simulink model "Transformation_dq_alphabeta_123_V1"  (R2022a)
settings: Solver=VariableStepAuto  StartTime=0.0  StopTime=0.2  RelTol=1e-3
InitFcn:
  | Ts_xadc = 0.1;
values from neighbouring files (symbols this model uses):
  f_c = 100000    [Trans_dq_alphabeta_123_params.m]
  T_50MHz = 1/f_50MHz    (= 2e-08)    [Trans_dq_alphabeta_123_params.m]
libraries: simulink x3
settings Model: DataTypeOverride=Off  Creator=trichte  LastModifiedBy=Andre Merx
settings SolverCC: AlgebraicLoopSolver=TrustRegion
settings DataIOCC: LimitDataPoints=on  SaveFormat=Array  SaveOutput=off  SaveTime=off  ReturnWorkspaceOutputs=off
settings OptimizationCC: BlockReduction=off  ConditionallyExecuteInputs=off  DefaultParameterBehavior=Inlined  LifeSpan=inf
settings DebuggingCC: AlgebraicLoopMsg=error  SolverPrmCheckMsg=warning  UnconnectedInputMsg=warning  UnconnectedOutputMsg=warning  UnconnectedLineMsg=warning  AllowSymbolicDim=off  StrictBusMsg=ErrorOnBusTreatedAsVector  SFUnexpectedBacktrackingDiag=warning  SFNoUnconditionalDefaultTransitionDiag=warning  SFExecutionAtInitializationDiag=none  SFMachineParentedDataDiag=warning  ArithmeticOperatorsInVariantConditions=warning
settings HardwareCC: ProdBitPerPointer=32  ProdBitPerSizeT=32  ProdBitPerPtrDiffT=32  ProdLargestAtomicFloat=None  ProdIntDivRoundTo=Undefined  ProdEndianess=Unspecified  ProdWordSize=32  ProdHWDeviceType=ASIC/FPGA->ASIC/FPGA  ProdEqTarget=off
settings ModelReferenceCC: PropagateSignalLabelsOutOfModel=off
settings SFSimCC: SimUseLocalCustomCode=off  CustomCodeUndefinedFunction=UseInterfaceOnly
settings RTWCC: RTWUseLocalCustomCode=off
settings CodeAppCC: StateflowObjectComments=on
settings GRTTargetCC: TargetLangStandard=C89/C90 (ANSI)
settings ConfigComp: CovMetricSettings=dw  CovSaveCumulativeToWorkspaceVar=on  CovSaveSingleToWorkspaceVar=on  CovExternalEMLEnable=off  CovSFcnEnable=off

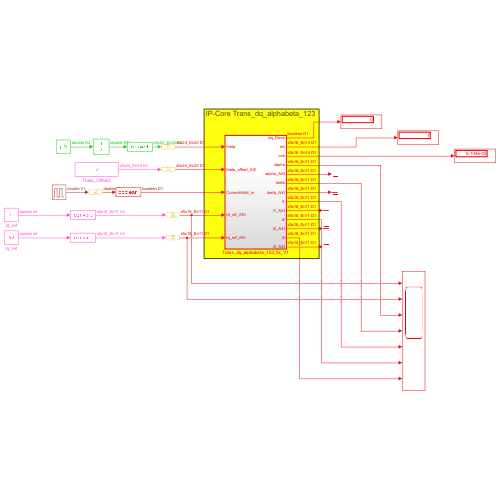
[thumbnail: Simulink's stored preview of the top-level diagram]
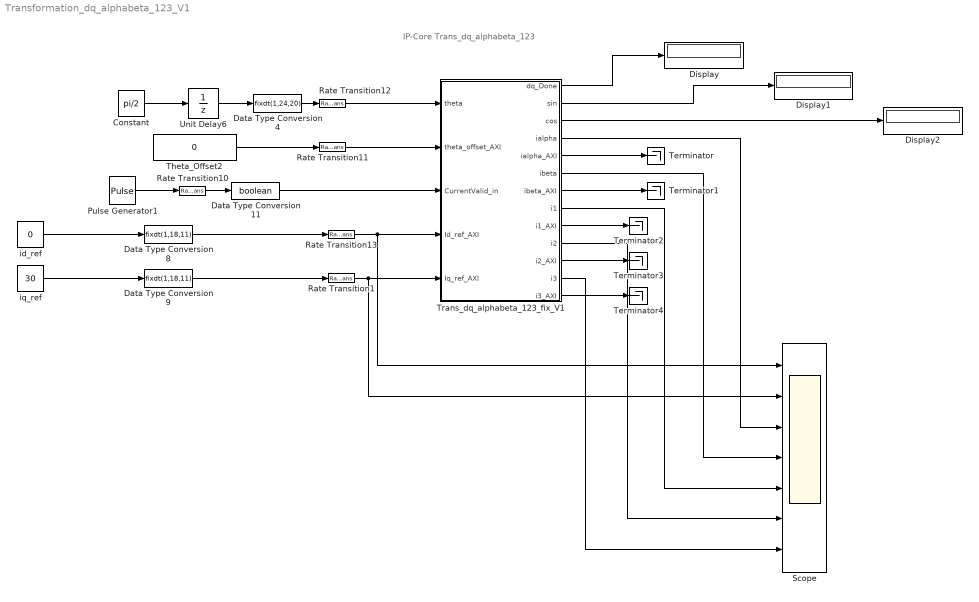
== system Transformation_dq_alphabeta_123_V1 ==
  note: IP-Core Trans_dq_alphabeta_123
  Constant : Constant  Value=pi/2  SampleTime=-1
  Data Type Conversion11 : DataTypeConversion  OutDataTypeStr=boolean  SaturateOnIntegerOverflow=off  RndMeth=Floor
  Data Type Conversion4 : DataTypeConversion  OutDataTypeStr=fixdt(1,24,20)  SaturateOnIntegerOverflow=off  RndMeth=Floor
  Data Type Conversion8 : DataTypeConversion  OutDataTypeStr=fixdt(1,18,11)  SaturateOnIntegerOverflow=off  RndMeth=Floor
  Data Type Conversion9 : DataTypeConversion  OutDataTypeStr=fixdt(1,18,11)  SaturateOnIntegerOverflow=off  RndMeth=Floor
  Display : Display
  Display1 : Display
  Display2 : Display
  Pulse Generator1 : DiscretePulseGenerator  PulseType=Time based  Period=1/f_c  PulseWidth=5
  Rate Transition{1,10..13} (5 alike) : RateTransition  OutPortSampleTime=T_50MHz
  Scope : Scope  NumInputPorts=7
  Terminator{,1..4} (5 alike) : Terminator
  Theta_Offset2 : Constant  Value=0  OutDataTypeStr=fixdt(1,24,20)
  Trans_dq_alphabeta_123_fix_V1 : Subsystem  TreatAsAtomicUnit=on
  Unit Delay6 : UnitDelay  SampleTime=1/f_c  HasFrameUpgradeWarning=on
  id_ref : Constant  Value=0
  iq_ref : Constant  Value=30
  wires:
  Theta_Offset2/1 -> Rate Transition11/1
  Data Type Conversion4/1 -> Rate Transition12/1
  Rate Transition1/1 -> Scope/2, Trans_dq_alphabeta_123_fix_V1/5(Iq_ref_AXI)
  Rate Transition11/1 -> Trans_dq_alphabeta_123_fix_V1/2(theta_offset_AXI)
  Data Type Conversion11/1 -> Trans_dq_alphabeta_123_fix_V1/3(CurrentValid_in)
  Rate Transition13/1 -> Scope/1, Trans_dq_alphabeta_123_fix_V1/4(Id_ref_AXI)
  Trans_dq_alphabeta_123_fix_V1/5(ialpha_AXI) -> Terminator/1
  Unit Delay6/1 -> Data Type Conversion4/1
  Data Type Conversion8/1 -> Rate Transition13/1
  Pulse Generator1/1 -> Rate Transition10/1
  Data Type Conversion9/1 -> Rate Transition1/1
  Trans_dq_alphabeta_123_fix_V1/13(i3_AXI) -> Terminator4/1
  Rate Transition12/1 -> Trans_dq_alphabeta_123_fix_V1/1(theta)
  Trans_dq_alphabeta_123_fix_V1/2(sin) -> Display1/1
  Trans_dq_alphabeta_123_fix_V1/11(i2_AXI) -> Terminator3/1
  Trans_dq_alphabeta_123_fix_V1/1(dq_Done) -> Display/1
  Trans_dq_alphabeta_123_fix_V1/6(ibeta) -> Scope/4
  Constant/1 -> Unit Delay6/1
  Trans_dq_alphabeta_123_fix_V1/9(i1_AXI) -> Terminator2/1
  Trans_dq_alphabeta_123_fix_V1/8(i1) -> Scope/5
  Trans_dq_alphabeta_123_fix_V1/3(cos) -> Display2/1
  id_ref/1 -> Data Type Conversion8/1
  iq_ref/1 -> Data Type Conversion9/1
  Rate Transition10/1 -> Data Type Conversion11/1
  Trans_dq_alphabeta_123_fix_V1/4(ialpha) -> Scope/3
  Trans_dq_alphabeta_123_fix_V1/7(ibeta_AXI) -> Terminator1/1
  Trans_dq_alphabeta_123_fix_V1/12(i3) -> Scope/7
  Trans_dq_alphabeta_123_fix_V1/10(i2) -> Scope/6

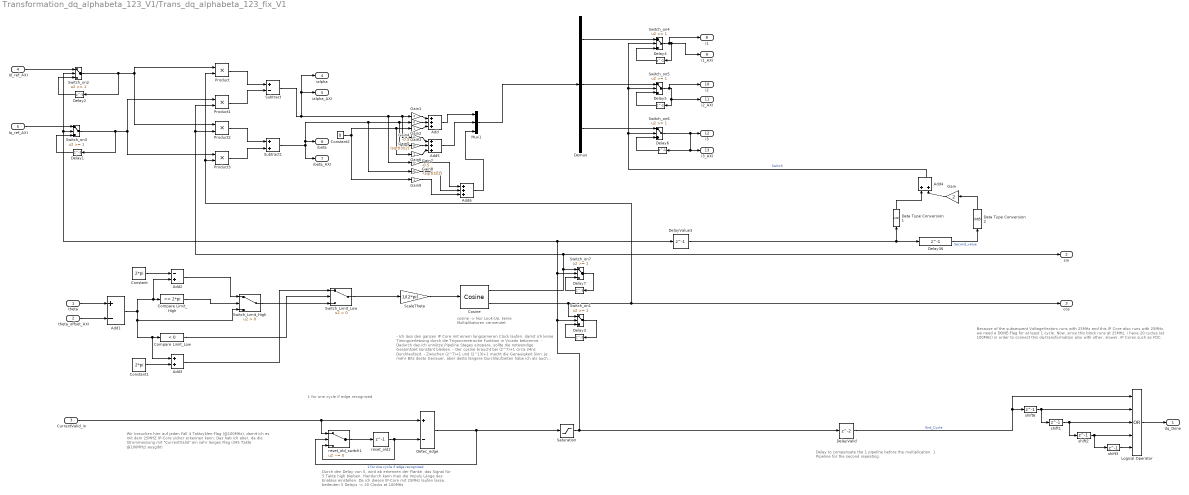
== system Transformation_dq_alphabeta_123_V1/Trans_dq_alphabeta_123_fix_V1 ==
  note: Delay to compensate the 1 pipeline before the multiplication.
      | 1 Pipeline for the second repeating.
  note: cosine -> Nur Look-Up,
      | keine Multiplikatoren
      | verwendet
  note: - Ich lass den ganzen IP Core mit einem langsameren Clock laufen,
      | damit ich keine Timingverletzung durch die Trigonometrische
      | Funktion in Vivado bekomme.
      | - Dadurch das ich unnütze Pipeline Stages einspare, sollte
      | die notwendige Gesamtzeit konstant bleiben.
      | - Der cosine braucht bei (2^7)+1 circa 24ns Durchlaufzeit.
      | - Zwischen (2^7)+1 und (2^13)+1 macht die Genauigkeit Sinn. Je mehr Bits
      | desto Genauer, aber desto längere Durchlaufzeiten habe ich als auch mehr
      | Ressourcen brauche ich. (Habe mich aktuell für (2^9)+1 entschieden.
  note: Durch den Delay von 5, wird ab erkennen der Flanke,
      |  das Signal für 5 Takte high bleiben.
      | Hierdurch kann man die Impuls Länge des Enables einstellen.
      | Da ich diesen IP-Core mit 25MHz laufen lasse, bedeuten 5 Delays -> 20 Clocks at 100MHz
  note: 1 for one cycle if edge recognized
  note: Wir brauchen hier auf jeden Fall 4 Taktzyklen-Flag (@100MHz),
      | damit ich es mit dem 25MHZ IP-Core sicher erkennen kann. Das hab
      | ich aber, da die Strommessung mit "CurrentValid" ein sehr langes Flag
      | (345 Takte @100MHz) ausgibt!
  note: Because of the subsequent VoltageVectors runs with 25MHz and this
      | IP Core also runs with 25MHz, we need a DONE-Flag for at least 1 cycle.
      | Now, since this block runs at 25MHz, i have 20 cycles (at 100MHz) in order
      | to connect this dq-transformation also with other, slower, IP Cores such as
      | FOC.
  theta : Inport
  theta_offset_AXI : Inport  Port=2
  CurrentValid_in : Inport  Port=3
  Id_ref_AXI : Inport  Port=4
  Iq_ref_AXI : Inport  Port=5
  Add : Sum  Inputs=+++  OutDataTypeStr=fixdt(1,18,11)
  Add1 : Sum  Inputs=+-  OutDataTypeStr=Inherit: Same as accumulator
  Add2 : Sum  Inputs=-+  OutDataTypeStr=Inherit: Same as first input
  Add3 : Sum  OutDataTypeStr=Inherit: Same as first input
  Add4 : Sum  AccumDataTypeStr=int8  OutDataTypeStr=int8  RndMeth=Simplest
  Add5 : Sum  Inputs=+++  OutDataTypeStr=fixdt(1,18,11)
  Add6 : Sum  Inputs=+++  OutDataTypeStr=fixdt(1,18,11)
  Compare Limit_High : simulink/Logic and Bit Operations/Compare To Constant  relop=>=  const=2*pi  OutDataTypeStr=boolean
  Compare Limit_Low : simulink/Logic and Bit Operations/Compare To Constant  relop=<  const=0  OutDataTypeStr=boolean
  Constant : Constant  Value=2*pi  OutDataTypeStr=fixdt(1,24,20)  SampleTime=T_50MHz
  Constant1 : Constant  Value=2*pi  OutDataTypeStr=fixdt(1,24,20)  SampleTime=T_50MHz
  Constant2 : Constant  Value=0  OutDataTypeStr=fixdt(1,18,11)  SampleTime=-1
  Cosine : simulink/Lookup Tables/Cosine  Formula=sin(2*pi*u) and cos(2*pi*u)  NumDataPoints=(2^9)+1  OutputWordLength=16  InternalRulePriority=Precision
      settings: SourceProductBaseCode=SL
  Data Type Conversion1 : DataTypeConversion  OutDataTypeStr=int8  SaturateOnIntegerOverflow=off  RndMeth=Floor
  Data Type Conversion2 : DataTypeConversion  OutDataTypeStr=int8  SaturateOnIntegerOverflow=off  RndMeth=Floor
  Delay{1..7,36} (8 alike) : Delay  DelayLength=1
  DelayValid : Delay
  DelayValue3 : Delay  DelayLength=1
  Demux : Demux  Outputs=3
  Detec_edge : Sum  Inputs=+-  AccumDataTypeStr=int8  OutDataTypeStr=int8
  Gain : Gain  Gain=2  RndMeth=Simplest
  Gain{1,3,6,9} (4 alike) : Gain  OutDataTypeStr=fixdt(1,18,11)
  Gain2 : Gain  Gain=0  OutDataTypeStr=fixdt(1,18,11)
  Gain4 : Gain  Gain=-0.5  OutDataTypeStr=fixdt(1,18,11)
  Gain5 : Gain  Gain=(sqrt(3)/2)  OutDataTypeStr=fixdt(1,18,11)
  Gain7 : Gain  Gain=-0.5  OutDataTypeStr=fixdt(1,18,11)
  Gain8 : Gain  Gain=-(sqrt(3)/2)  OutDataTypeStr=fixdt(1,18,11)
  Logical Operator : Logic  Operator=OR  Inputs=5  AllPortsSameDT=off  OutDataTypeStr=boolean
  Mux1 : Mux  Inputs=3
  Product{,1..3} (4 alike) : Product  OutDataTypeStr=fixdt(1,18,11)
  Saturation : Saturate  UpperLimit=1  LowerLimit=0  OutMin=[0]  OutMax=[1]  OutDataTypeStr=fixdt(0,1)
  ScaleTheta : Gain  Gain=1/(2*pi)  OutDataTypeStr=Inherit: Same as input
  Subtract : Sum  Inputs=+-  OutDataTypeStr=fixdt(1,18,11)
  Subtract1 : Sum  OutDataTypeStr=fixdt(1,18,11)
  Switch_Limit_High : Switch  Criteria=u2 > Threshold  OutDataTypeStr=fixdt(1,24,20)  SaturateOnIntegerOverflow=off  InputSameDT=off
  Switch_Limit_Low : Switch  Criteria=u2 > Threshold  OutDataTypeStr=fixdt(1,24,20)  SaturateOnIntegerOverflow=off  InputSameDT=off
  Switch_on1 : Switch  Threshold=1  OutDataTypeStr=fixdt(1,16,14)  SaturateOnIntegerOverflow=off  InputSameDT=off
  Switch_on{2..6} (5 alike) : Switch  Threshold=1  OutDataTypeStr=Inherit: Inherit via back propagation  RndMeth=Simplest  SaturateOnIntegerOverflow=off  InputSameDT=off
  Switch_on7 : Switch  Threshold=1  OutDataTypeStr=fixdt(1,16,14)  SaturateOnIntegerOverflow=off  InputSameDT=off
  reset_old2 : Delay  DelayLength=1
  reset_old_switch1 : Switch  Criteria=u2 ~= 0  SaturateOnIntegerOverflow=off  InputSameDT=off
  shift{1..3,6} (4 alike) : Delay  DelayLength=1
  dq_Done : Outport  VectorParamsAs1DForOutWhenUnconnected=off
  sin : Outport  Port=2  VectorParamsAs1DForOutWhenUnconnected=off
  cos : Outport  Port=3  VectorParamsAs1DForOutWhenUnconnected=off
  ialpha : Outport  Port=4  VectorParamsAs1DForOutWhenUnconnected=off
  ialpha_AXI : Outport  Port=5  VectorParamsAs1DForOutWhenUnconnected=off
  ibeta : Outport  Port=6  VectorParamsAs1DForOutWhenUnconnected=off
  ibeta_AXI : Outport  Port=7  VectorParamsAs1DForOutWhenUnconnected=off
  i1 : Outport  Port=8  VectorParamsAs1DForOutWhenUnconnected=off
  i1_AXI : Outport  Port=9  VectorParamsAs1DForOutWhenUnconnected=off
  i2 : Outport  Port=10  VectorParamsAs1DForOutWhenUnconnected=off
  i2_AXI : Outport  Port=11  VectorParamsAs1DForOutWhenUnconnected=off
  i3 : Outport  Port=12  VectorParamsAs1DForOutWhenUnconnected=off
  i3_AXI : Outport  Port=13  VectorParamsAs1DForOutWhenUnconnected=off
  wires:
  theta/1 -> Add1/1
  Add1/1 -> Add2/2, Compare Limit_High/1, Switch_Limit_High/3, Add3/1, Compare Limit_Low/1
  theta_offset_AXI/1 -> Add1/2
  Switch_Limit_High/1 -> Switch_Limit_Low/3
  Compare Limit_High/1 -> Switch_Limit_High/2
  Compare Limit_Low/1 -> Switch_Limit_Low/2
  Constant/1 -> Add2/1
  Add2/1 -> Switch_Limit_High/1
  Constant1/1 -> Add3/2
  Add3/1 -> Switch_Limit_Low/1
  Saturation/1 -> DelayValid/1, Switch_on1/2, Switch_on7/2, Switch_on2/2, Switch_on3/2, DelayValue3/1
  Delay3/1 -> Switch_on1/3
  Delay7/1 -> Switch_on7/3
  ScaleTheta/1 -> Cosine/1
  Switch_on7/1 -> Delay7/1
  Switch_on1/1 -> Delay3/1
  Detec_edge/1 -> Saturation/1, reset_old_switch1/2  "1 for one cycle if edge recognized"
  reset_old2/1 -> reset_old_switch1/3, Detec_edge/2
  CurrentValid_in/1 -> reset_old_switch1/1, Detec_edge/1
  reset_old_switch1/1 -> reset_old2/1
  DelayValid/1 -> shift6/1, Logical Operator/1  "End_Cycle"
  shift6/1 -> Logical Operator/2, shift1/1
  Logical Operator/1 -> dq_Done/1
  DelayValue3/1 -> Data Type Conversion1/1, Delay36/1
  Data Type Conversion1/1 -> Add4/1
  Gain/1 -> Add4/2
  Delay36/1 -> Data Type Conversion2/1  "Second_value"
  Data Type Conversion2/1 -> Gain/1
  shift1/1 -> Logical Operator/3, shift2/1
  shift2/1 -> shift3/1, Logical Operator/4
  shift3/1 -> Logical Operator/5
  Id_ref_AXI/1 -> Switch_on2/1
  Delay2/1 -> Switch_on2/3
  Delay1/1 -> Switch_on3/3
  Iq_ref_AXI/1 -> Switch_on3/1
  Constant2/1 -> Gain9/1, Gain6/1, Gain3/1
  Demux/1 -> Switch_on4/1
  Switch_on4/1 -> i1_AXI/1, Delay4/1, i1/1
  Delay4/1 -> Switch_on4/3
  Delay5/1 -> Switch_on5/3
  Switch_on5/1 -> i2/1, i2_AXI/1, Delay5/1
  Demux/2 -> Switch_on5/1
  Delay6/1 -> Switch_on6/3
  Switch_on6/1 -> i3/1, i3_AXI/1, Delay6/1
  Demux/3 -> Switch_on6/1
  Gain1/1 -> Add/1
  Gain2/1 -> Add/2
  Gain3/1 -> Add/3
  Add/1 -> Mux1/1
  Gain5/1 -> Add5/2
  Gain4/1 -> Add5/1
  Gain6/1 -> Add5/3
  Add5/1 -> Mux1/2
  Gain8/1 -> Add6/2
  Gain7/1 -> Add6/1
  Gain9/1 -> Add6/3
  Add6/1 -> Mux1/3
  Add4/1 -> Switch_on6/2, Switch_on5/2, Switch_on4/2  "Switch"
  Mux1/1 -> Demux/1
  Switch_Limit_Low/1 -> ScaleTheta/1
  Subtract/1 -> Gain7/1, Gain4/1, Gain1/1, ialpha/1, ialpha_AXI/1
  Subtract1/1 -> Gain8/1, Gain5/1, Gain2/1, ibeta/1, ibeta_AXI/1
  Product1/1 -> Subtract/2
  Product2/1 -> Subtract1/1
  Product/1 -> Subtract/1
  Switch_on3/1 -> Delay1/1, Product1/1, Product3/1
  Switch_on2/1 -> Delay2/1, Product/1, Product2/1
  Product3/1 -> Subtract1/2
  Cosine/1 -> sin/1, Product2/2, Product1/2, Switch_on7/1
  Cosine/2 -> cos/1, Product3/2, Product/2, Switch_on1/1
